simulink model "Square_nest sowing"  (R2018b)
settings: Solver=FixedStepAuto  StartTime=0.0  StopTime=inf  FixedStep=0.001  MaxStep=0.001  MinStep=0.0001  RelTol=1e-4  AbsTol=1e-5  EnableMultiTasking=on
model workspace (MAT data in the model file):
  Enk = 1200
libraries: fl_lib x6, nesl_utility x5, elec_lib x1
settings Model: PauseTimes=2  Creator=Admin  LastModifiedBy=Admin
settings SolverCC: AutoInsertRateTranBlk=on  InsertRTBMode=Always
settings DataIOCC: SaveFormat=Array  SaveState=on  SignalLogging=off  InspectSignalLogs=on  LoggingToFile=on

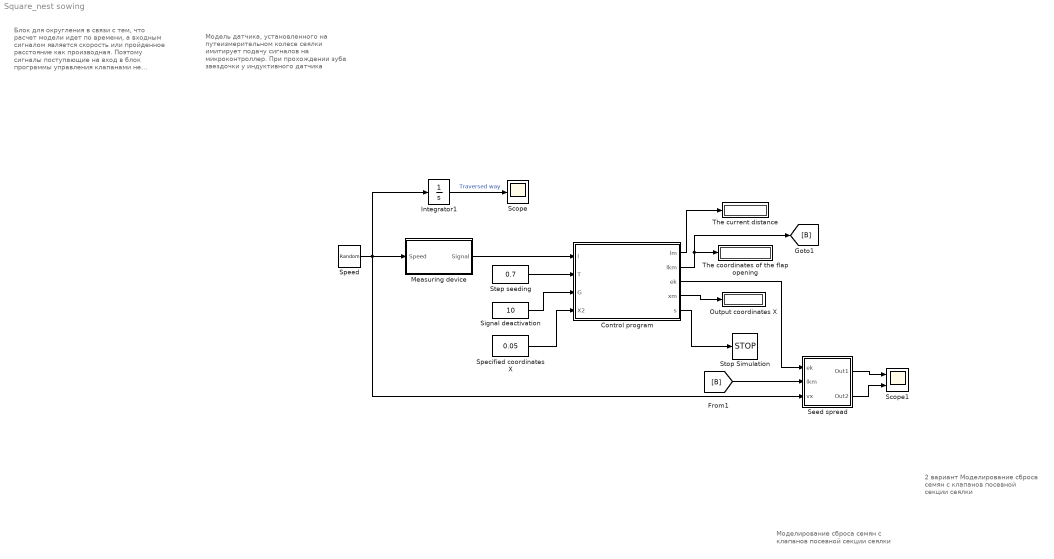
== system Square_nest sowing ==
  note: Моделирование сброса семян с клапанов посевной секции сеялки
  note: Модель датчика, установленного на
      | путеизмерительном колесе сеялки
      | имитирует подачу сигналов на микроконтроллер. При прохождении зуба звездочки у индуктивного датчика
  note: Блок для округления
      | в связи с тем, что расчет модели идет по времени, а входным сигналом является скорость или пройденное расстояние как производная. Поэтому сигналы поступающие на вход в блок программы управления клапанами не соотвтетствует шагу расчета модели и следовательно возникает рассоглосование
  note: 2 вариант Моделирование сброса семян с клапанов посевной секции сеялки
  Integrator1 : Integrator
  Measuring device : Subsystem
  Output coordinates Х : Display
      settings: Format=bank
  Scope : Scope
  Scope1 : Scope  NumInputPorts=2
  Seed spread : Subsystem
  Signal deactivation : Constant  Value=10
  "Specified coordinates X " : Constant  Value=0.05  VectorParams1D=off
  Speed : RandomNumber  Mean=2.5  Variance=0.3  SampleTime=0.1
  Step seeding : Constant  Value=0.7
  Stop Simulation : Stop
  The coordinates of the flap opening : Display
      settings: Format=bank
  The current distance : Display
      settings: Format=bank
  Сontrol program : MATLAB Function  TreatAsAtomicUnit=on
  wires:
  Step seeding/1 -> Сontrol program/2(T)
  Сontrol program/5(s) -> Stop Simulation/1
  Сontrol program/3(ek) -> Seed spread/1(ek)
  Integrator1/1 -> Scope/1  "Traversed way"
  Сontrol program/2(lkm) -> The coordinates of the flap opening/1, [B]
  Measuring device/1("Signal ") -> Сontrol program/1(l)
  Сontrol program/1(lm) -> The current distance/1
  "Specified coordinates X "/1 -> Сontrol program/4(X2)
  Signal deactivation/1 -> Сontrol program/3(G)
  Сontrol program/4(xm) -> Output coordinates Х/1
  [B] -> Seed spread/2(lkm)
  Seed spread/1(Out1) -> Scope1/1
  Seed spread/2(Out2) -> Scope1/2
  Speed/1 -> Integrator1/1, Seed spread/3(vx), Measuring device/1(Speed)

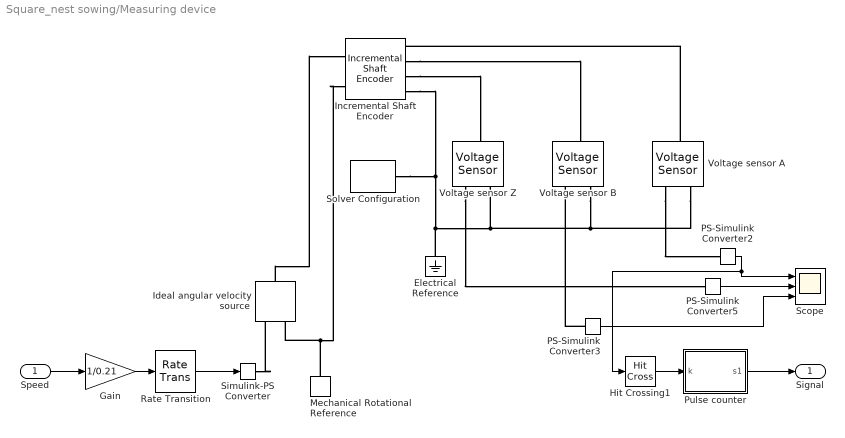
== system Square_nest sowing/Measuring device ==
  Speed : Inport
  Electrical Reference : fl_lib/Electrical/Electrical Elements/Electrical Reference
  Gain : Gain  Gain=1/0.21
  Hit Crossing1 : HitCross  HitCrossingOffset=0.6  HitCrossingDirection=rising
  Ideal angular velocity source : fl_lib/Mechanical/Mechanical Sources/Ideal Angular Velocity Source
  Incremental Shaft Encoder : elec_lib/Sensors/Incremental Shaft Encoder  NPulse=213  Vm=1 V  angle0=0 rad
      settings: SourceProductName=Simscape Electronics  SourceProductBaseCode=SN
  Mechanical Rotational Reference : fl_lib/Mechanical/Rotational Elements/Mechanical Rotational Reference
  PS-Simulink Converter2 : nesl_utility/PS-Simulink Converter  PhysicalDomain=network_engine_domain  SubClassName=ps_output  LeftPortType=input  RightPortType=output  PseudoPeriodic=off  Frequencies=[]  Unit=1  AffineConversion=off
  PS-Simulink Converter3 : nesl_utility/PS-Simulink Converter  PhysicalDomain=network_engine_domain  SubClassName=ps_output  LeftPortType=input  RightPortType=output  PseudoPeriodic=off  Frequencies=[]  Unit=1  AffineConversion=off
  PS-Simulink Converter5 : nesl_utility/PS-Simulink Converter  PhysicalDomain=network_engine_domain  SubClassName=ps_output  LeftPortType=input  RightPortType=output  PseudoPeriodic=off  Frequencies=[]  Unit=1  AffineConversion=off
  Pulse counter : MATLAB Function  TreatAsAtomicUnit=on
  Rate Transition : RateTransition
  Scope : Scope  NumInputPorts=3
  Simulink-PS Converter : nesl_utility/Simulink-PS Converter  PhysicalDomain=network_engine_domain  SubClassName=ps_input  LeftPortType=input  RightPortType=output  PseudoPeriodic=off  Frequencies=[]  NoiseDistribution=none  NoiseParameters=[]  Unit=rad/s  AffineConversion=off  FilteringAndDerivatives=provide  SimscapeFilterOrder=1  InputFilterTimeConstant=0.001  UdotUserProvided=0
  Solver Configuration : nesl_utility/Solver Configuration  PhysicalDomain=network_engine_domain  SubClassName=solver  LeftPortType=input  RightPortType=generic  Tones=[]  Harmonics=[]  SimulateNoise=off  Profile=off  UseLocalSampling=off  EnableSwitchedLinearOptims=on  FrequencyDomain=off  UseCCode=off  RelTol=0.001  AbsTol=1e-06  MinStep=1e-09  ToWorkspace=off  RevertToSquareIcSolve=off  NumHomotopyIterations=100  PhasorMode=off  PhasorModeNumHarmonics=1  DoDC=off  ResidualTolerance=1e-09  UseLocalSolver=off  LocalSolverChoice=NE_BACKWARD_EULER_ADVANCER  LocalSolverSampleTime=0.001  DoFixedCost=off  MaxNonlinIter=3  MaxModeIter=2  LinearAlgebra=auto  EquationFormulation=NE_TIME_EF  DelaysMemoryBudget=1024  AutomaticFiltering=on  FilteringTimeConstant=0.001  PartitionStorageMethod=AS_NEEDED  PartitionMemoryBudget=1024
  Voltage sensor A : fl_lib/Electrical/Electrical Sensors/Voltage Sensor
  Voltage sensor B : fl_lib/Electrical/Electrical Sensors/Voltage Sensor
  Voltage sensor Z : fl_lib/Electrical/Electrical Sensors/Voltage Sensor
  "Signal " : Outport
  wires:
  PS-Simulink Converter3/1 -> Scope/3
  PS-Simulink Converter2/1 -> Hit Crossing1/1, Scope/1
  Pulse counter/1(s1) -> "Signal "/1
  PS-Simulink Converter5/1 -> Scope/2
  Hit Crossing1/1 -> Pulse counter/1("k ")
  Gain/1 -> Rate Transition/1
  Rate Transition/1 -> Simulink-PS Converter/1
  Speed/1 -> Gain/1
  connections:
  Voltage sensor A/LConn1 -- Incremental Shaft Encoder/RConn1
  Incremental Shaft Encoder/RConn4 -- Electrical Reference/LConn1 -- Voltage sensor A/RConn2 -- Voltage sensor B/RConn2 -- Voltage sensor Z/RConn2 -- Solver Configuration/RConn1
  Voltage sensor A/RConn1 -- PS-Simulink Converter2/LConn1
  Simulink-PS Converter/RConn1 -- Ideal angular velocity source/RConn1
  PS-Simulink Converter3/LConn1 -- Voltage sensor B/RConn1
  Ideal angular velocity source/LConn1 -- Incremental Shaft Encoder/LConn1
  Incremental Shaft Encoder/LConn2 -- Mechanical Rotational Reference/LConn1 -- Ideal angular velocity source/RConn2
  Voltage sensor Z/RConn1 -- PS-Simulink Converter5/LConn1
  Incremental Shaft Encoder/RConn3 -- Voltage sensor Z/LConn1
  Incremental Shaft Encoder/RConn2 -- Voltage sensor B/LConn1

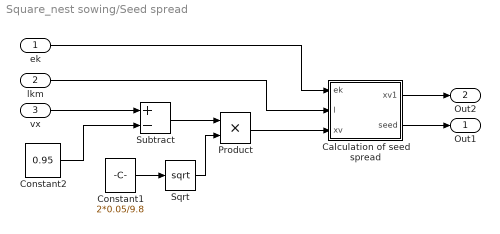
== system Square_nest sowing/Seed spread ==
  ek : Inport
  lkm : Inport  Port=2
  vx : Inport  Port=3
  Calculation of seed spread : MATLAB Function  TreatAsAtomicUnit=on
  Constant1 : Constant  Value=2*0.05/9.8  VectorParams1D=off
  Constant2 : Constant  Value=0.95  VectorParams1D=off
  Product : Product
  Sqrt : Sqrt  SaturateOnIntegerOverflow=on
  Subtract : Sum  Inputs=+-
  Out1 : Outport
  Out2 : Outport  Port=2
  wires:
  Sqrt/1 -> Product/2
  Constant1/1 -> Sqrt/1
  Calculation of seed spread/2(seed) -> Out1/1
  Calculation of seed spread/1(xv1) -> Out2/1
  Product/1 -> Calculation of seed spread/3(xv)
  ek/1 -> Calculation of seed spread/1(ek)
  lkm/1 -> Calculation of seed spread/2(l)
  vx/1 -> Subtract/1
  Subtract/1 -> Product/1
  Constant2/1 -> Subtract/2

== matlab function Square_nest sowing/Seed spread/Calculation of seed spread ==
  settings: updateMethod=DISCRETE
  data: ek input; xv1 output; l input; seed output; xv input
function [xv1,seed] = fcn(ek,l,xv)
seed=0;

persistent vx
if isempty(vx)  
    vx = 0;
end


persistent k
if isempty(k)  
    k = 1;
end

persistent j
if isempty(j)  
    j = 0;
end

persistent m
if isempty(m)  
    m = 0;
end

persistent n1
if isempty(n1)  
    n1 = 0;
end


if ek==1
    m=l+xv;
    k=k+1;
    vx=xv;
end

if l>=m & l~=0 & k>j
    seed=1;
    n1=n1+1;
    j=j+1;
end

xv1=vx;
% seed;
n=n1;

== matlab function Square_nest sowing/Measuring device/Pulse counter ==
  settings: updateMethod=DISCRETE
  data: k input; s1 output
function s1  = fcn(k)

persistent s
if isempty(s)  
    s = 0;
end 

persistent n
if isempty(n)  
    n = 0;
end

if k>0
    s=s+1;
    n=s*2*pi*0.21/213;
    k;
   
else
    n
end

y=n
s1=s

== matlab function Square_nest sowing/Сontrol program ==
  settings: updateMethod=DISCRETE
  data: lm output; l input; lkm output; ek output; T input; xm output; s output; G input; X2 input
function [lm, lkm, ek, xm, s] = fcn(l, T, G, X2)

%инициализация переменной для остановки программы управления
 % (симуляция выключения измерительного устройства - энкодера) 
 % измерительного устройства по сигналу спутника
s=0; 

% моделирование сигнала октрытия электроклапанов на исп. механизм.      
ek=0;        

% определение переводного коэффициента kf (расстояние за 1 сигнал энкодера)
kf=2*pi*0.21/213; 

% перевод из метров в количество сигналов 
t=round(T/kf);
g=round(G/kf);

% перевод сигналов, поступающих из энкодера в метры
lm=l*kf;

% инициализация входных переменных
% локальные персистентные переменные
persistent n  % кол-во откр. клапан. за один проход
persistent lk  % расстояние на котором сработали клапаны
persistent x  % расстояние отк. клап. в начале 1 и последующих проходов

if isempty(n)  
    n = 0;
end
    
if isempty(lk)
    lk = 0;
end

if isempty(x)
    x = round(X2/kf); %количество сигналов с энкодера;
end

% Запуск работы эл. клапанов.
if l==x
   lk=l;
   lkm=lk*kf;
   ek=1;  % откр. электроклапаны
   n=n+1; % кол-во открытия электроклапанов

%сравнение текущей позиции сеялки с шагом посева    
elseif l-lk == t 
   lk=l;
   lkm=lk*kf;
   ek=1;  % откр. электроклапаны
   n=n+1; % кол-во открытия электроклапанов

% симуляция выключения измерительного устройства   
elseif l >= g 
   x= l-lk; % запись расстояния последнего срабатывния клапанов на проходе.
   s=1; % отправка сигнала на блок STOP
end

% Вывод показателей работы и сигналов в симулинк:
n1=n
lkm=lk*kf;
xm=x*kf;
